simulink model "CLoopsim"  (R2023a)
settings: Solver=VariableStepAuto  StartTime=0.0  StopTime=10.0  RelTol=1e-3
libraries: cstblocks x2
settings Model: Creator=brucekj  LastModifiedBy=brucekj

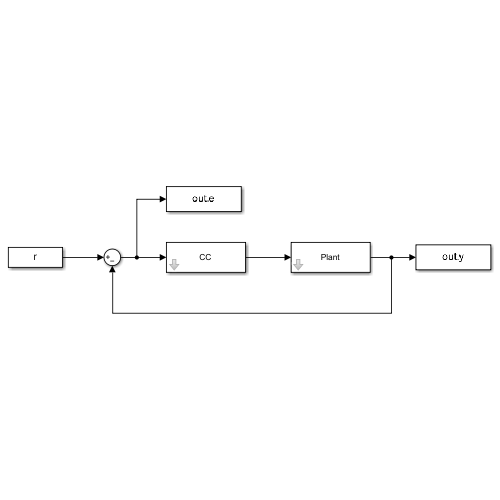
[thumbnail: Simulink's stored preview of the top-level diagram]
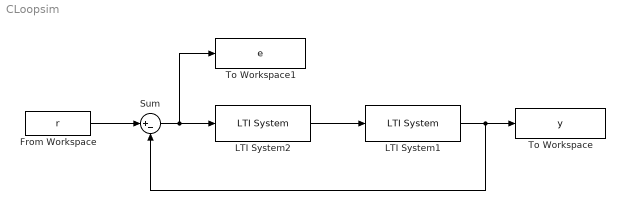
== system CLoopsim ==
  From Workspace : FromWorkspace  VariableName=r  SampleTime=0.001
  LTI System1 : cstblocks/LTI System  sys=Plant  IC=[]
  LTI System2 : cstblocks/LTI System  sys=CC  IC=[]
  Sum : Sum  Inputs=|+-
  To Workspace : ToWorkspace  VariableName=y  SaveFormat=Timeseries  SampleTime=-1
  To Workspace1 : ToWorkspace  VariableName=e  SaveFormat=Timeseries  SampleTime=-1
  wires:
  From Workspace/1 -> Sum/1
  Sum/1 -> To Workspace1/1, LTI System2/1
  LTI System2/1 -> LTI System1/1
  LTI System1/1 -> Sum/2, To Workspace/1
